simulink model "SimplifiedModel"  (R2022a)
settings: Solver=VariableStepAuto  StartTime=0.0  StopTime=1000  RelTol=1e-3
values from neighbouring files (symbols this model uses):
  a1 = 0.45    [init.m]
  A1 = 154    [init.m]
  a2 = 0.25    [init.m]
  g = 980.665    [init.m]
  H1_max = 100    [init.m]
  Q1_max = 100    [init.m]
  s12 = 0.5    [init.m]
  s23 = s12    (= 0.5)    [init.m]
libraries: dspnetwork x4
settings Model: Creator=Dottorandi  LastModifiedBy=marco
settings SolverCC: AlgebraicLoopSolver=TrustRegion
settings DataIOCC: ReturnWorkspaceOutputs=off
settings DebuggingCC: UnconnectedInputMsg=warning  UnconnectedOutputMsg=warning  UnconnectedLineMsg=warning  SFMachineParentedDataDiag=warning  ArithmeticOperatorsInVariantConditions=warning
settings SFSimCC: SimUseLocalCustomCode=off  CustomCodeUndefinedFunction=UseInterfaceOnly
settings RTWCC: RTWUseLocalCustomCode=off

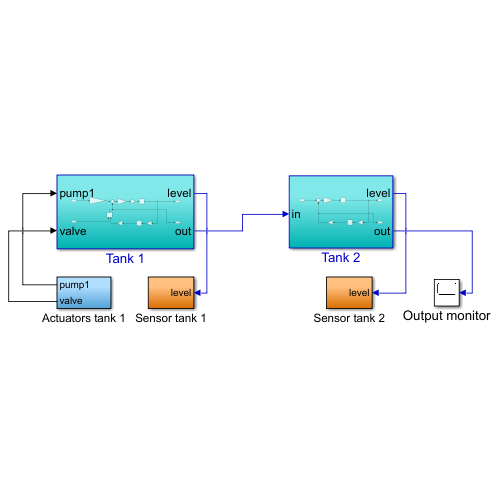
[thumbnail: Simulink's stored preview of the top-level diagram]
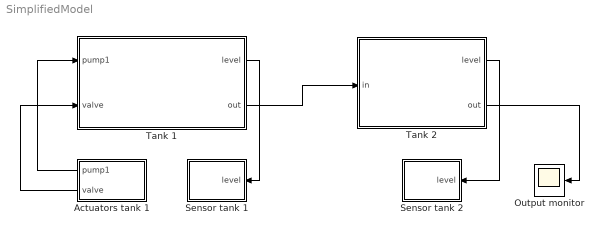
== system SimplifiedModel ==
  Actuators tank 1 : Subsystem
  Output monitor : Scope
  Sensor tank 1 : Subsystem
  Sensor tank 2 : Subsystem
  Tank 1 : Subsystem
  Tank 2 : Subsystem
  wires:
  Tank 1/2(out) -> Tank 2/1(in)
  Tank 2/2(out) -> Output monitor/1
  Tank 1/1(level) -> Sensor tank 1/1(level)
  Actuators tank 1/1(pump1) -> Tank 1/1(pump1)
  Actuators tank 1/2(valve) -> Tank 1/2(valve)
  Tank 2/1(level) -> Sensor tank 2/1(level)

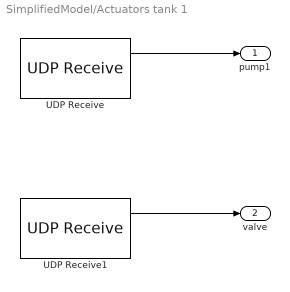
== system SimplifiedModel/Actuators tank 1 ==
  UDP Receive : dspnetwork/UDP Receive  localURL='0.0.0.0'  localPort=10003  remoteURL='0.0.0.0'  remotePort=-1  recvBufferSize=2  dims=1  signalDatatype=uint16  isComplex=off  isVarSize=off  showBlockingTime=on  blockingTime=0  sampletime=1  blockPlatform=LINUX
  UDP Receive1 : dspnetwork/UDP Receive  localURL='0.0.0.0'  localPort=10003  remoteURL='0.0.0.0'  remotePort=-1  recvBufferSize=2  dims=1  signalDatatype=uint16  isComplex=off  isVarSize=off  showBlockingTime=on  blockingTime=0  sampletime=1  blockPlatform=LINUX
  pump1 : Outport  VectorParamsAs1DForOutWhenUnconnected=off
  valve : Outport  Port=2  VectorParamsAs1DForOutWhenUnconnected=off
  wires:
  UDP Receive1/1 -> valve/1
  UDP Receive/1 -> pump1/1

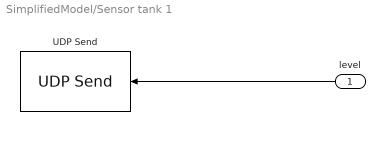
== system SimplifiedModel/Sensor tank 1 ==
  level : Inport
  UDP Send : dspnetwork/UDP Send  remoteURL='localhost'  remotePort=10001  localURL='255.255.255.255'  localPortSource=Automatically determine  localPort=-1  sendBufferSize=8192  sampletime=-1  blockPlatform=LINUX  separateLengthPort=0
  wires:
  level/1 -> UDP Send/1

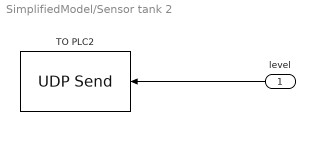
== system SimplifiedModel/Sensor tank 2 ==
  level : Inport
  TO PLC2 : dspnetwork/UDP Send  remoteURL='localhost'  remotePort=10001  localURL='255.255.255.255'  localPortSource=Automatically determine  localPort=-1  sendBufferSize=8192  sampletime=-1  blockPlatform=LINUX  separateLengthPort=0
  wires:
  level/1 -> TO PLC2/1

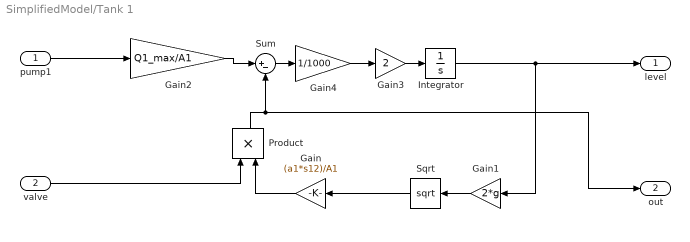
== system SimplifiedModel/Tank 1 ==
  pump1 : Inport
  valve : Inport  Port=2
  Gain : Gain  Gain=(a1*s12)/A1
  Gain1 : Gain  Gain=2*g
  Gain2 : Gain  Gain=Q1_max/A1
  Gain3 : Gain  Gain=2
  Gain4 : Gain  Gain=1/1000
  Integrator : Integrator  InitialCondition=0.11*H1_max
  Product : Product
  Sqrt : Sqrt
  Sum : Sum  Inputs=|+-
  level : Outport  VectorParamsAs1DForOutWhenUnconnected=off
  out : Outport  Port=2  VectorParamsAs1DForOutWhenUnconnected=off
  wires:
  pump1/1 -> Gain2/1
  Integrator/1 -> Gain1/1, level/1
  Sum/1 -> Gain4/1
  Gain/1 -> Product/2
  Sqrt/1 -> Gain/1
  Gain1/1 -> Sqrt/1
  valve/1 -> Product/1
  Product/1 -> out/1, Sum/2
  Gain2/1 -> Sum/1
  Gain3/1 -> Integrator/1
  Gain4/1 -> Gain3/1

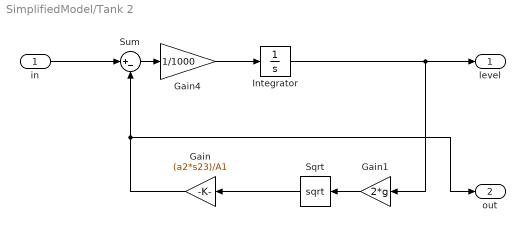
== system SimplifiedModel/Tank 2 ==
  in : Inport
  Gain : Gain  Gain=(a2*s23)/A1
  Gain1 : Gain  Gain=2*g
  Gain4 : Gain  Gain=1/1000
  Integrator : Integrator  InitialCondition=0.11*H1_max
  Sqrt : Sqrt
  Sum : Sum  Inputs=|+-
  level : Outport  VectorParamsAs1DForOutWhenUnconnected=off
  out : Outport  Port=2  VectorParamsAs1DForOutWhenUnconnected=off
  wires:
  in/1 -> Sum/1
  Integrator/1 -> Gain1/1, level/1
  Sum/1 -> Gain4/1
  Sqrt/1 -> Gain/1
  Gain1/1 -> Sqrt/1
  Gain/1 -> out/1, Sum/2
  Gain4/1 -> Integrator/1
